simulink model "QEI_Model_2016a"  (R2020a)
settings: Solver=VariableStepAuto  StartTime=0.0  StopTime=6  MaxStep=0.001  RelTol=1e-3  EnableMultiTasking=on
values from neighbouring files (symbols this model uses):
  deltaP = 35.714285*10^-6    (= 3.5714285e-05)    [Incremental_Encoder.m]
  J = 33.3 *10^-7+ ((1/121) *0.5* 28.65*10^-6)    (= 3.44838842975e-06)    [Incremental_Encoder.m]
  k_M = 1/(466)    (= 0.00214592274678)    [Incremental_Encoder.m]
  RM = 0.21    [Incremental_Encoder.m]
  T_QEI = 0.001    [Incremental_Encoder.m]
libraries: fl_lib x6, nesl_utility x5, dspswit3 x4, simulink x3, powerlib_meascontrol x2, simulink_extras x1, ee_lib x1, dspsrcs4 x1
settings Model: Creator=sebastianfriedrich  LastModifiedBy=sebastianfriedrich
settings DataIOCC: ExternalInput=test_vel  ReturnWorkspaceOutputs=off
settings OptimizationCC: LifeSpan=inf
settings DebuggingCC: SFUnexpectedBacktrackingDiag=warning  SFNoUnconditionalDefaultTransitionDiag=warning  SFExecutionAtInitializationDiag=none  ArithmeticOperatorsInVariantConditions=warning
settings SFSimCC: SimUseLocalCustomCode=off  CustomCodeUndefinedFunction=UseInterfaceOnly
settings RTWCC: RTWUseLocalCustomCode=off
settings CodeAppCC: StateflowObjectComments=on
settings GRTTargetCC: TargetLangStandard=C89/C90 (ANSI)
settings ConfigComp: CovMetricSettings=dw  CovHtmlReporting=on  CovSaveCumulativeToWorkspaceVar=on  CovSaveSingleToWorkspaceVar=on  CovExternalEMLEnable=off
settings SimscapeCC: SimscapeNormalizeSystem=off

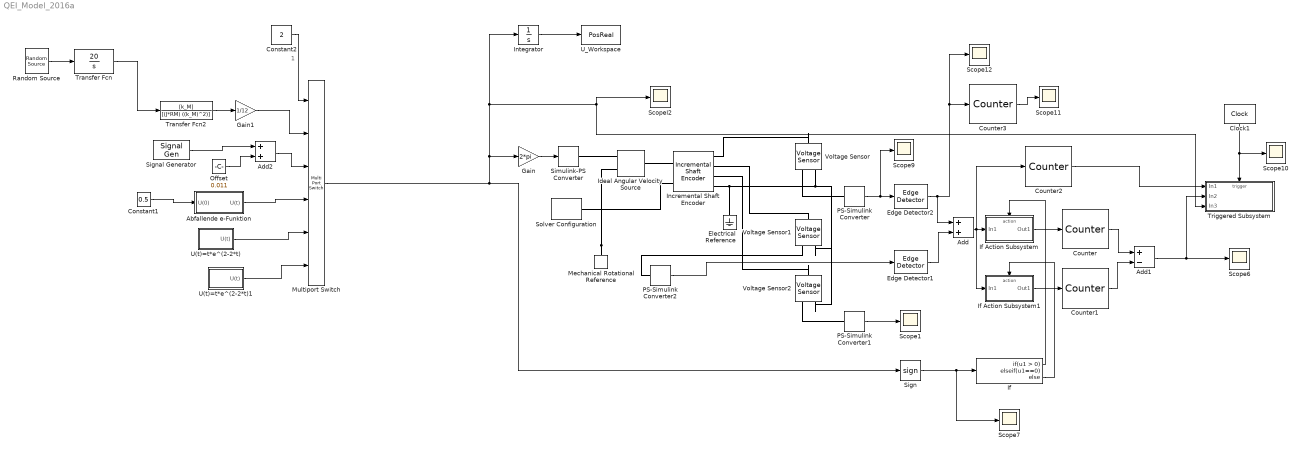
== system QEI_Model_2016a ==
  note: 1
  Abfallende e-Funktion : Subsystem
  Add : Sum
  Add1 : Sum  Inputs=+-
  Add2 : Sum
  Clock1 : simulink_extras/Flip Flops/Clock  period=T_QEI
  Constant1 : Constant  Value=0.5
  Constant2 : Constant  Value=2
  Counter{,1..3} (4 alike) : dspswit3/Counter  Direction=Up  CountEvent=Rising edge  CounterSize=32 bits  MaxCount=255  InitialCount=0  Output=Count  HitValue=32  ResetInput=off  SamplesPerFrame=1  Ts=1  CntDtype=double  HitDtype=Logical
  Edge Detector1 : powerlib_meascontrol/Logic/Edge Detector  model=Either  ic=0  Ts=0
      settings: SourceProductBaseCode=PS
  Edge Detector2 : powerlib_meascontrol/Logic/Edge Detector  model=Either  ic=0  Ts=0
      settings: SourceProductBaseCode=PS
  Electrical Reference : fl_lib/Electrical/Electrical Elements/Electrical Reference
  Gain : Gain  Gain=2*pi
  Gain1 : Gain  Gain=1/12
  Ideal Angular Velocity Source : fl_lib/Mechanical/Mechanical Sources/Ideal Angular Velocity Source
  If : If  ElseIfExpressions=u1==0
  If Action Subsystem : Subsystem  TreatAsAtomicUnit=on
  If Action Subsystem1 : Subsystem  TreatAsAtomicUnit=on
  Incremental Shaft Encoder : ee_lib/Sensors & Transducers/Incremental Shaft Encoder  NPulse=7000  Vm=5 V  angle0=0 deg
      settings: SourceProductBaseCode=PS  InternalSimscapePortConfiguration="{\"Bottom\":[],\"Left\":[{\"id\":\"R\",\"label\":\"R\",\"type\":\"foundation.mechanical.rotational.rotational\"},{\"id\":\"C\",\"label\":\"C\",\"type\":\"foundation.mechanical.rotational.rotational\"}],\"Right\":[{\"id\":\"A\",\"label\":\"A\",\"type\":\"foundation.electrical.electrical\"},{\"id\":\"B\",\"label\":\"B\",\"type\":\"foundation.electrical.electrical\"},{\"id\":\"Z\",\"label\":\"Z\",\"type\":\"foundation.electrical.electrical\"},{\"id\":\"GND\",\"label\":\"REF\",\"type\":\"foundation.electrical.electrical\"}],\"Top\":[]}"
  Integrator : Integrator
  Mechanical Rotational Reference : fl_lib/Mechanical/Rotational Elements/Mechanical Rotational Reference
  Multiport Switch : MultiPortSwitch  Inputs=5
  Offset : Constant  Value=0.011
  PS-Simulink Converter : nesl_utility/PS-Simulink Converter  PhysicalDomain=network_engine_domain  SubClassName=ps_output  LeftPortType=input  RightPortType=output  PseudoPeriodic=off  Frequencies=[]  Unit=1  AffineConversion=off
  PS-Simulink Converter1 : nesl_utility/PS-Simulink Converter  PhysicalDomain=network_engine_domain  SubClassName=ps_output  LeftPortType=input  RightPortType=output  PseudoPeriodic=off  Frequencies=[]  Unit=1  AffineConversion=off
  PS-Simulink Converter2 : nesl_utility/PS-Simulink Converter  PhysicalDomain=network_engine_domain  SubClassName=ps_output  LeftPortType=input  RightPortType=output  PseudoPeriodic=off  Frequencies=[]  Unit=1  AffineConversion=off
  Random Source : dspsrcs4/Random Source  SrcType=Uniform  NormMethod=Ziggurat  CltLength=12  MinVal=-0.22  MaxVal=0.22  MeanVal=0  VarVal=1  RepMode=Not repeatable  rawSeed=1  IsInherit=off  SampMode=Continuous  SampTime=1  SampFrame=1  DataType=Double  OutComplex=Real  OutputFrames=off
  Scope{1,6..7,9..12} (7 alike) : Scope
  ScopeI2 : Scope
  Sign : Signum
  Signal Generator : SignalGenerator  WaveForm=square  Amplitude=0.011  Frequency=2*pi/4  Units=rad/sec
  Simulink-PS Converter : nesl_utility/Simulink-PS Converter  PhysicalDomain=network_engine_domain  SubClassName=ps_input  LeftPortType=input  RightPortType=output  PseudoPeriodic=off  Frequencies=[]  NoiseDistribution=none  NoiseParameters=[]  Unit=rad/s  AffineConversion=off  FilteringAndDerivatives=zero  SimscapeFilterOrder=1  InputFilterTimeConstant=0.001  UdotUserProvided=1
  Solver Configuration : nesl_utility/Solver Configuration  PhysicalDomain=network_engine_domain  SubClassName=solver  LeftPortType=input  RightPortType=generic  Tones=[]  Harmonics=[]  SimulateNoise=off  Profile=off  UseLocalSampling=off  EnableSwitchedLinearOptims=on  FrequencyDomain=off  UseCCode=off  RelTol=0.001  AbsTol=1e-06  MinStep=1e-09  ToWorkspace=off  RevertToSquareIcSolve=off  NumHomotopyIterations=100  PhasorMode=off  PhasorModeNumHarmonics=1  DoDC=off  ResidualTolerance=1e-09  UseLocalSolver=off  LocalSolverChoice=NE_BACKWARD_EULER_ADVANCER  LocalSolverSampleTime=0.001  DoFixedCost=off  MaxNonlinIter=3  MaxModeIter=2  LinearAlgebra=Sparse  EquationFormulation=NE_TIME_EF  DelaysMemoryBudget=1024  AutomaticFiltering=on  FilteringTimeConstant=0.001  PartitionStorageMethod=AS_NEEDED  PartitionMemoryBudget=1024  PartitionMethod=FAST
  Transfer Fcn : TransferFcn  Numerator=[20]  Denominator=[1 0]
  Transfer Fcn2 : TransferFcn  Numerator=[k_M]  Denominator=[(J*RM) ((k_M)^2)]
  Triggered Subsystem : Subsystem  TreatAsAtomicUnit=on
  U(t)=t*e^(2-2*t) : Subsystem
  U(t)=t*e^(2-2*t)1 : Subsystem
  U_Workspace : ToWorkspace  VariableName=PosReal  SaveFormat=Structure With Time  SampleTime=-1
  Voltage Sensor : fl_lib/Electrical/Electrical Sensors/Voltage Sensor
  Voltage Sensor1 : fl_lib/Electrical/Electrical Sensors/Voltage Sensor
  Voltage Sensor2 : fl_lib/Electrical/Electrical Sensors/Voltage Sensor
  wires:
  PS-Simulink Converter/1 -> Scope9/1, Edge Detector2/1
  PS-Simulink Converter1/1 -> Scope1/1
  PS-Simulink Converter2/1 -> Edge Detector1/1
  Edge Detector2/1 -> Scope12/1, Counter3/1, Add/1
  Edge Detector1/1 -> Add/2
  Sign/1 -> Scope7/1, If/1
  If/1 -> If Action Subsystem/Action
  Add/1 -> Counter2/1, If Action Subsystem/1(In1), If Action Subsystem1/1(In1)
  If Action Subsystem/1(Out1) -> Counter/1
  If/3 -> If Action Subsystem1/Action
  If Action Subsystem1/1(Out1) -> Counter1/1
  Counter/1 -> Add1/1
  Counter1/1 -> Add1/2
  Add1/1 -> Triggered Subsystem/2(In2), Scope6/1
  Clock1/1 -> Scope10/1, Triggered Subsystem/Trigger
  Gain/1 -> Simulink-PS Converter/1
  Counter3/1 -> Scope11/1
  Constant1/1 -> Abfallende e-Funktion/1(U(0))
  Constant2/1 -> Multiport Switch/1
  Abfallende e-Funktion/1(U(t)) -> Multiport Switch/4
  U(t)=t*e^(2-2*t)/1(U(t)) -> Multiport Switch/5
  Counter2/1 -> Triggered Subsystem/1(In1)
  U(t)=t*e^(2-2*t)1/1(U(t)) -> Multiport Switch/6
  Signal Generator/1 -> Add2/1
  Offset/1 -> Add2/2
  Integrator/1 -> U_Workspace/1
  Add2/1 -> Multiport Switch/3
  Gain1/1 -> Multiport Switch/2
  Random Source/1 -> Transfer Fcn/1
  Transfer Fcn2/1 -> Gain1/1
  Transfer Fcn/1 -> Transfer Fcn2/1
  Multiport Switch/1 -> ScopeI2/1, Triggered Subsystem/3(In3), Integrator/1, Gain/1, Sign/1
  connections:
  Mechanical Rotational Reference/LConn1 -- Incremental Shaft Encoder/LConn2 -- Ideal Angular Velocity Source/RConn2 -- Solver Configuration/RConn1
  Incremental Shaft Encoder/RConn4 -- Electrical Reference/LConn1 -- Voltage Sensor/RConn2 -- Voltage Sensor2/RConn2 -- Voltage Sensor1/RConn2
  Voltage Sensor/LConn1 -- Incremental Shaft Encoder/RConn1
  Voltage Sensor/RConn1 -- PS-Simulink Converter/LConn1
  Incremental Shaft Encoder/RConn2 -- Voltage Sensor1/LConn1
  Voltage Sensor2/LConn1 -- Incremental Shaft Encoder/RConn3
  PS-Simulink Converter1/LConn1 -- Voltage Sensor2/RConn1
  Voltage Sensor1/RConn1 -- PS-Simulink Converter2/LConn1
  Ideal Angular Velocity Source/RConn1 -- Simulink-PS Converter/RConn1
  Ideal Angular Velocity Source/LConn1 -- Incremental Shaft Encoder/LConn1

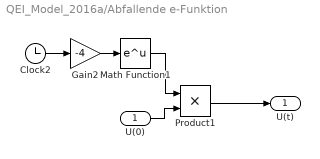
== system QEI_Model_2016a/Abfallende e-Funktion ==
  U(0) : Inport
  Clock2 : Clock
  Gain2 : Gain  Gain=-4
  Math Function1 : Math  SignedPower=on  SaturateOnIntegerOverflow=on
  Product1 : Product
  U(t) : Outport
  wires:
  Clock2/1 -> Gain2/1
  Gain2/1 -> Math Function1/1
  Math Function1/1 -> Product1/1
  U(0)/1 -> Product1/2
  Product1/1 -> U(t)/1

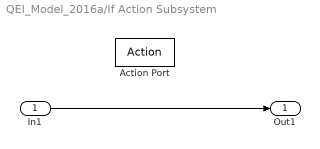
== system QEI_Model_2016a/If Action Subsystem ==
  In1 : Inport
  Action Port : ActionPort  ActionPortLabel=if(u1 > 0)
  Out1 : Outport
  wires:
  In1/1 -> Out1/1

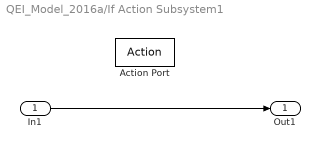
== system QEI_Model_2016a/If Action Subsystem1 ==
  In1 : Inport
  Action Port : ActionPort  ActionPortLabel=else
  Out1 : Outport
  wires:
  In1/1 -> Out1/1

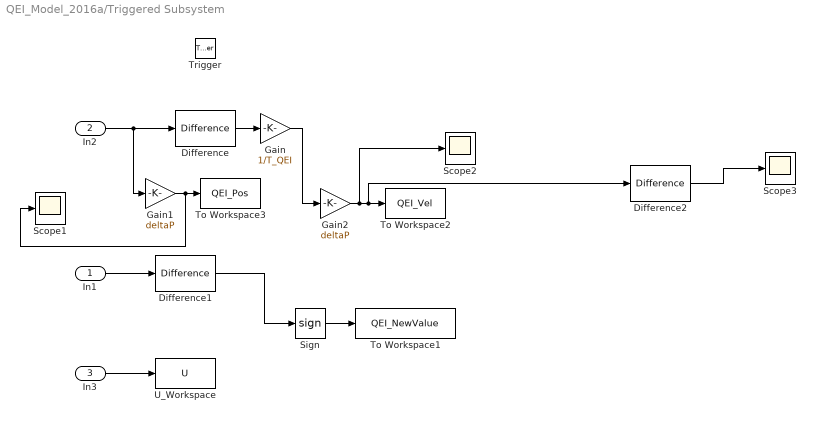
== system QEI_Model_2016a/Triggered Subsystem ==
  In1 : Inport
  In2 : Inport  Port=2
  In3 : Inport  Port=3
  Trigger : TriggerPort  VariantControl=Variant
  Difference : simulink/Discrete/Difference  ICPrevInput=0.0  OutMin=[]  OutMax=[]  OutDataType=fixdt(1, 16)  OutScaling=2^-10  DoSatur=off
  Difference1 : simulink/Discrete/Difference  ICPrevInput=0.0  OutMin=[]  OutMax=[]  OutDataType=fixdt(1, 16)  OutScaling=2^-10  DoSatur=off
  Difference2 : simulink/Discrete/Difference  ICPrevInput=0.0  OutMin=[]  OutMax=[]  OutDataType=fixdt(1, 16)  OutScaling=2^-10  DoSatur=off
  Gain : Gain  Gain=1/T_QEI
  Gain1 : Gain  Gain=deltaP
  Gain2 : Gain  Gain=deltaP
  Scope1 : Scope
  Scope2 : Scope
  Scope3 : Scope
  Sign : Signum
  To Workspace1 : ToWorkspace  VariableName=QEI_NewValue  SaveFormat=Structure With Time  SampleTime=-1
  To Workspace2 : ToWorkspace  VariableName=QEI_Vel  SaveFormat=Structure With Time  SampleTime=-1
  To Workspace3 : ToWorkspace  VariableName=QEI_Pos  SaveFormat=Structure With Time  SampleTime=-1
  U_Workspace : ToWorkspace  VariableName=U  SaveFormat=Structure With Time  SampleTime=-1
  wires:
  In2/1 -> Difference/1, Gain1/1
  Difference/1 -> Gain/1
  Gain/1 -> Gain2/1
  Gain1/1 -> Scope1/1, To Workspace3/1
  Gain2/1 -> Scope2/1, Difference2/1, To Workspace2/1
  In1/1 -> Difference1/1
  Sign/1 -> To Workspace1/1
  Difference1/1 -> Sign/1
  In3/1 -> U_Workspace/1
  Difference2/1 -> Scope3/1

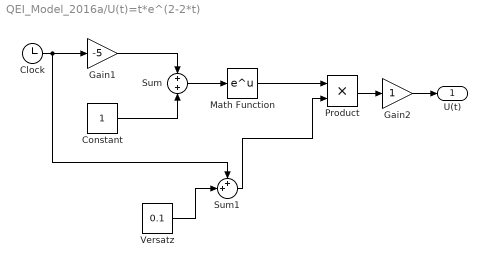
== system QEI_Model_2016a/U(t)=t*e^(2-2*t) ==
  Clock : Clock
  Constant : Constant
  Gain1 : Gain  Gain=-5
  Gain2 : Gain
  Math Function : Math  SignedPower=on  SaturateOnIntegerOverflow=on
  Product : Product
  Sum : Sum  Inputs=+|+
  Sum1 : Sum  Inputs=++|
  Versatz : Constant  Value=0.1
  U(t) : Outport
  wires:
  Clock/1 -> Sum1/1, Gain1/1
  Math Function/1 -> Product/1
  Gain1/1 -> Sum/1
  Constant/1 -> Sum/2
  Sum/1 -> Math Function/1
  Product/1 -> Gain2/1
  Versatz/1 -> Sum1/2
  Sum1/1 -> Product/2
  Gain2/1 -> U(t)/1

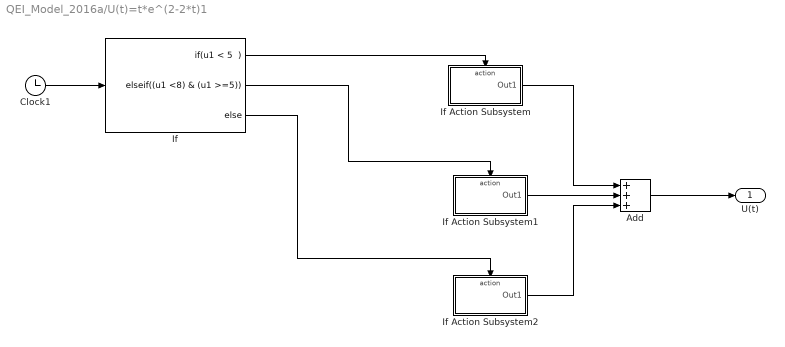
== system QEI_Model_2016a/U(t)=t*e^(2-2*t)1 ==
  Add : Sum  Inputs=+++
  Clock1 : Clock
  If : If  IfExpression=u1 < 5  ElseIfExpressions=(u1 <8) & (u1 >=5)
  If Action Subsystem : Subsystem  TreatAsAtomicUnit=on
  If Action Subsystem1 : Subsystem  TreatAsAtomicUnit=on
  If Action Subsystem2 : Subsystem  TreatAsAtomicUnit=on
  U(t) : Outport
  wires:
  Clock1/1 -> If/1
  If/1 -> If Action Subsystem/Action
  If/2 -> If Action Subsystem1/Action
  If/3 -> If Action Subsystem2/Action
  If Action Subsystem/1(Out1) -> Add/1
  If Action Subsystem1/1(Out1) -> Add/2
  If Action Subsystem2/1(Out1) -> Add/3
  Add/1 -> U(t)/1

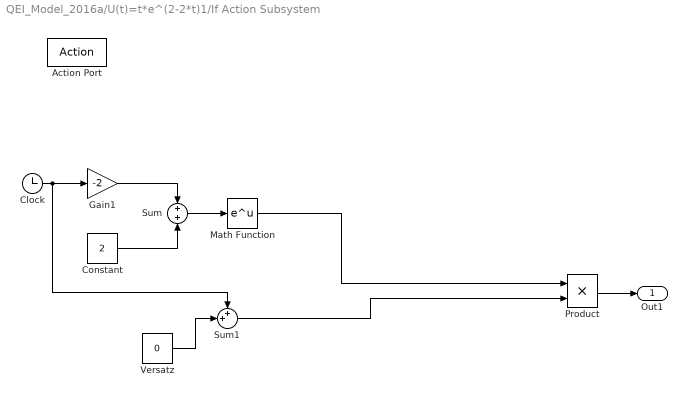
== system QEI_Model_2016a/U(t)=t*e^(2-2*t)1/If Action Subsystem ==
  Action Port : ActionPort  ActionPortLabel="if(u1 < 5  )"
  Clock : Clock
  Constant : Constant  Value=2
  Gain1 : Gain  Gain=-2
  Math Function : Math  SignedPower=on  SaturateOnIntegerOverflow=on
  Product : Product
  Sum : Sum  Inputs=+|+
  Sum1 : Sum  Inputs=++|
  Versatz : Constant  Value=0
  Out1 : Outport
  wires:
  Clock/1 -> Sum1/1, Gain1/1
  Math Function/1 -> Product/1
  Gain1/1 -> Sum/1
  Constant/1 -> Sum/2
  Sum/1 -> Math Function/1
  Product/1 -> Out1/1
  Versatz/1 -> Sum1/2
  Sum1/1 -> Product/2

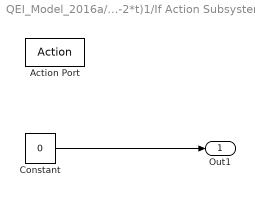
== system QEI_Model_2016a/U(t)=t*e^(2-2*t)1/If Action Subsystem1 ==
  Action Port : ActionPort  ActionPortLabel=elseif((u1 <8) & (u1 >=5))
  Constant : Constant  Value=0
  Out1 : Outport
  wires:
  Constant/1 -> Out1/1

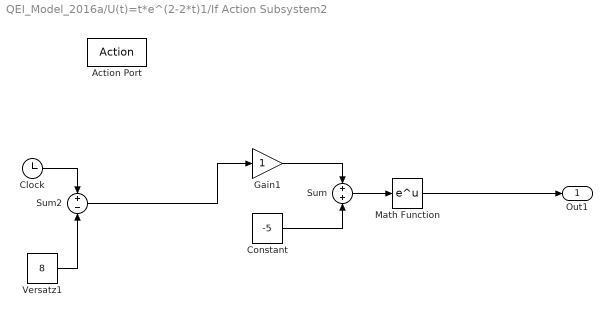
== system QEI_Model_2016a/U(t)=t*e^(2-2*t)1/If Action Subsystem2 ==
  Action Port : ActionPort  ActionPortLabel=else
  Clock : Clock
  Constant : Constant  Value=-5
  Gain1 : Gain
  Math Function : Math  SignedPower=on  SaturateOnIntegerOverflow=on
  Sum : Sum  Inputs=+|+
  Sum2 : Sum  Inputs=+|-
  Versatz1 : Constant  Value=8
  Out1 : Outport
  wires:
  Math Function/1 -> Out1/1
  Sum2/1 -> Gain1/1
  Gain1/1 -> Sum/1
  Constant/1 -> Sum/2
  Sum/1 -> Math Function/1
  Clock/1 -> Sum2/1
  Versatz1/1 -> Sum2/2
